simulink model "LAB1"  (R2020a)
settings: Solver=VariableStepAuto  StartTime=0.0  StopTime=0.006  MaxStep=0.000001  RelTol=1e-3
settings Model: Creator=danie  LastModifiedBy=danie

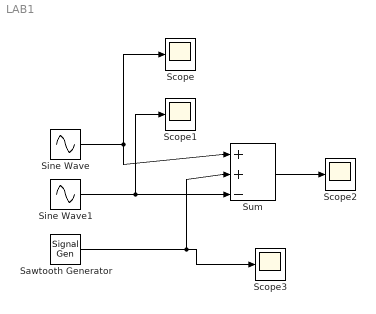
== system LAB1 ==
  Sawtooth Generator : SignalGenerator  WaveForm=sawtooth  Amplitude=-3  Frequency=1000*2*pi  Units=rad/sec
  Scope{,1..3} (4 alike) : Scope
  Sine Wave : Sin  Amplitude=4  Frequency=1000*2*pi  SampleTime=0
  Sine Wave1 : Sin  Amplitude=5  Frequency=1000*2*pi  Phase=pi/4  SampleTime=0
  Sum : Sum  Inputs=|++-
  wires:
  Sine Wave/1 -> Sum/1, Scope/1
  Sine Wave1/1 -> Sum/3, Scope1/1
  Sum/1 -> Scope2/1
  Sawtooth Generator/1 -> Sum/2, Scope3/1
